simulink model "Shading_Fuzzy_single_phase_inverter"  (R2025a)
settings: Solver=ode23tb  StartTime=0.0  StopTime=2  FixedStep=1e-8  MaxStep=1e-5  RelTol=1e-4
values from neighbouring files (symbols this model uses):
  init_duty = 0.5    [generate_final_results.m]    (also in master_eval.m; params.m)
  sample_time_FLC = 0.005    [generate_final_results.m]    (also in master_eval.m; params.m)
  sample_time_mv_avg = 1e-4    (= 0.0001)    [generate_final_results.m]    (also in master_eval.m; params.m)
  temp = 25    [data_gen.m]    (also in generate_final_results.m; master_eval.m; params.m; shade_no_shade_graphs.m)
undefined symbols (not defined in the file or in its folder): DiscIntNeverNeededParam, irr
libraries: spsMosfetLib x5, spsSeriesRLCBranchLib x5, eeGeneralControl x3, spsCurrentMeasurementLib x2, spsFirstOrderFilterLib x2, slpidlib x2, simulink x2, spsVoltageMeasurementLib x2, spsACVoltageSourceLib x1, spsAlphaBetaZerotodq0Lib x1, spsDiodeLib x1, fuzblock x1
settings Model: Creator=gayathri  LastModifiedBy=harsh

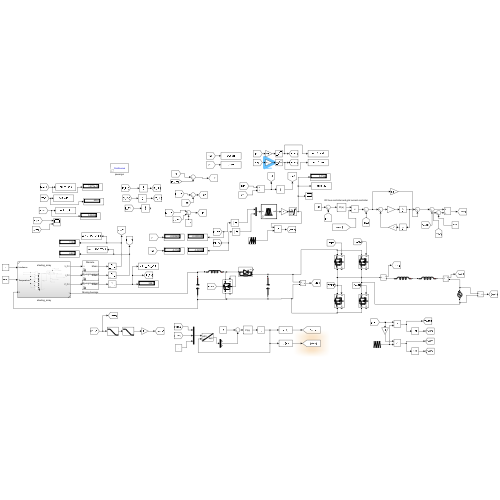
[thumbnail: Simulink's stored preview of the top-level diagram]
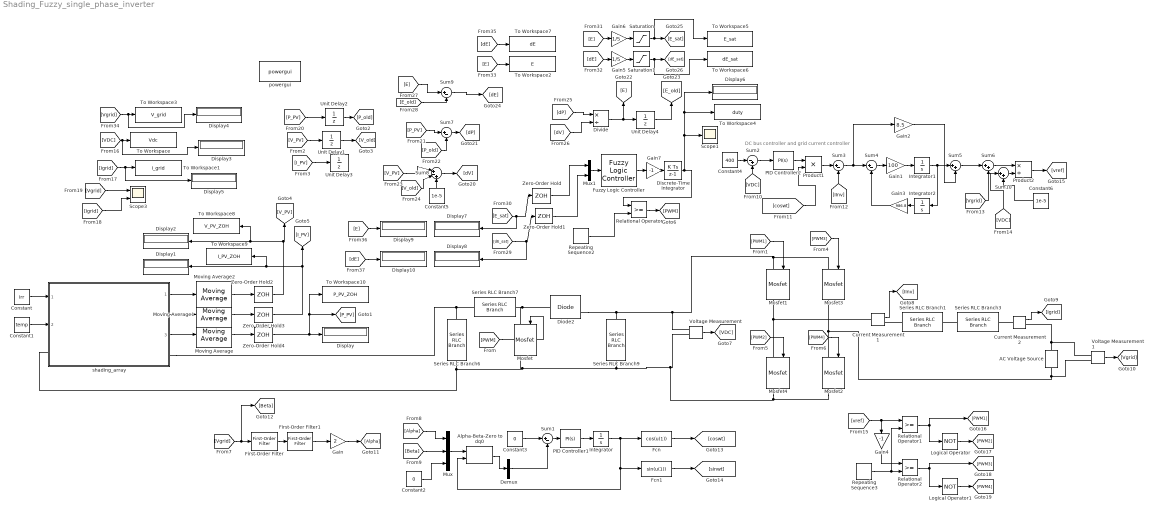
== system Shading_Fuzzy_single_phase_inverter ==
  note: DC bus controller and grid current controller
  AC Voltage Source : spsACVoltageSourceLib/AC Voltage Source  Amplitude=325  Phase=0  Frequency=50  SampleTime=0  Measurements=None  BusType=swing  Pref=10e3  Qref=0  Qmin=-inf  Qmax=+inf
  Alpha-Beta-Zero to dq0 : spsAlphaBetaZerotodq0Lib/Alpha-Beta-Zero to dq0  Alignment=90 degrees behind phase A axis
  Constant : Constant  Value=irr
  Constant1 : Constant  Value=temp
  Constant2 : Constant  Value=0
  Constant3 : Constant  Value=0
  Constant4 : Constant  Value=400
  Constant5 : Constant  Value=1e-5
  Constant6 : Constant  Value=1e-5
  Current Measurement1 : spsCurrentMeasurementLib/Current Measurement  PhasorSimulation=off  OutputType=Complex  PSBequivalent=0
  Current Measurement2 : spsCurrentMeasurementLib/Current Measurement  PhasorSimulation=off  OutputType=Complex  PSBequivalent=0
  Demux : Demux  Outputs=3
  Diode2 : spsDiodeLib/Diode  Ron=0.001  Lon=0  Vf=0.8  IC=0  UseSnubber=0  Rs=500  Cs=250e-9  Measurements=on
  Discrete-Time Integrator : DiscreteIntegrator  InitialCondition=init_duty  SampleTime=sample_time_FLC  LimitOutput=on  UpperSaturationLimit=0.9  LowerSaturationLimit=0.1  ICPrevOutput=DiscIntNeverNeededParam  ICPrevScaledInput=DiscIntNeverNeededParam
  Display{,1..10} (11 alike) : Display
  Divide : Product  Inputs=*/
  Fcn : Fcn  Expr=cos(u(1))
  Fcn1 : Fcn  Expr=sin(u(1))
  First-Order Filter : spsFirstOrderFilterLib/First-Order Filter  FilterType=Lowpass  Tc=1/(2*pi*50)  Ts=0  Initialize=off  Vac_Init=[0, 0, 60]  Vdc_Init=0  PlotResponse=off  FreqRange="[0,  200,  1]"
  First-Order Filter1 : spsFirstOrderFilterLib/First-Order Filter  FilterType=Lowpass  Tc=1/(2*pi*50)  Ts=0  Initialize=off  Vac_Init=[0, 0, 60]  Vdc_Init=0  PlotResponse=off  FreqRange="[0,  200,  1]"
  Fuzzy Logic Controller : fuzblock/Fuzzy Logic  Controller  FIS='fuzzy_mppt.fis'  OutputSampleNumber=101  DataType=double  UseLookupTable=off  NumBreakpoints=10  FuzzifiedInputs=off  RuleFiringStrengths=off  RuleOutputs=off  AggregatedOutputs=off  SimulateUsing=Interpreted execution  OutOfRangeInputValueMessage=warning  NoRuleFiredMessage=warning  EmptyOutputFuzzySetMessage=warning
  Gain : Gain  Gain=2
  Gain1 : Gain  Gain=100
  Gain2 : Gain  Gain=8.5
  Gain3 : Gain  Gain=986.8
  Gain4 : Gain  Gain=-1
  Gain5 : Gain  Gain=1/5
  Gain6 : Gain  Gain=1/5
  Gain7 : Gain  Gain=-1
  Integrator : Integrator
  Integrator1 : Integrator
  Integrator2 : Integrator
  Logical Operator : Logic  Operator=NOT  AllPortsSameDT=off  OutDataTypeStr=boolean
  Logical Operator1 : Logic  Operator=NOT  AllPortsSameDT=off  OutDataTypeStr=boolean
  Mosfet{,1..4} (5 alike) : spsMosfetLib/Mosfet  Ron=0.1  Lon=0  Rd=0.01  Vfd=0  IC=0  Rs=1e5  Cs=inf  Measurements=on
  Moving Average : eeGeneralControl/Moving Average  VariantControl=Variant1  LabelModeActiveChoice=Discrete  f=100  x0=0  BufferSize=8192  Ts=sample_time_mv_avg
      settings: LibrarySourceBlock=ee_sl_lib/General Control/Moving Average
  Moving Average1 : eeGeneralControl/Moving Average  VariantControl=Variant1  LabelModeActiveChoice=Discrete  f=100  x0=0  BufferSize=8192  Ts=sample_time_mv_avg
      settings: LibrarySourceBlock=ee_sl_lib/General Control/Moving Average
  Moving Average2 : eeGeneralControl/Moving Average  VariantControl=Variant1  LabelModeActiveChoice=Discrete  f=100  x0=0  BufferSize=8192  Ts=sample_time_mv_avg
      settings: LibrarySourceBlock=ee_sl_lib/General Control/Moving Average
  Mux : Mux  Inputs=3
  Mux1 : Mux  Inputs=2
  PID Controller1 : slpidlib/PID Controller  Controller=PI  Form=Parallel  TimeDomain=Continuous-time  UseExternalTs=off  SampleTime=-1  IntegratorMethod=Forward Euler  FilterMethod=Forward Euler  ControllerParametersSource=internal  P=10  I=5000  UseKiTs=off  D=0  UseExternalDerivativeSource=off  N=100  UseFilter=on  TunerSelectOption=Transfer Function Based (PID Tuner App)  InitialConditionSource=internal  InitialConditionForIntegrator=0  InitialConditionForFilter=0  DifferentiatorICPrevScaledInput=0  ExternalReset=none  TrackingMode=off  Kt=1  LimitOutput=off  SatLimitsSource=internal  UpperSaturationLimit=inf  LowerSaturationLimit=-inf  LinearizeAsGain=on  AntiWindupMode=none  Kb=1  LimitIntegrator=off  UpperIntegratorSaturationLimit=inf  LowerIntegratorSaturationLimit=-inf  POutMin=[]  POutMax=[]  IOutMin=[]  IOutMax=[]  DOutMin=[]  DOutMax=[]  NOutMin=[]  NOutMax=[]  SumOutMin=[]  SumOutMax=[]  SaturationOutMin=[]  SaturationOutMax=[]  PParamMin=[]  PParamMax=[]  IParamMin=[]  IParamMax=[]  DParamMin=[]  DParamMax=[]  NParamMin=[]  NParamMax=[]  KbParamMin=[]  KbParamMax=[]  KtParamMin=[]  KtParamMax=[]  KbOutMin=[]  KbOutMax=[]  KtOutMin=[]  KtOutMax=[]  IntegratorOutMin=[]  IntegratorOutMax=[]  FilterOutMin=[]  FilterOutMax=[]  SumI1OutMin=[]  SumI1OutMax=[]  SumI2OutMin=[]  SumI2OutMax=[]  SumI3OutMin=[]  SumI3OutMax=[]  SumI4OutMin=[]  SumI4OutMax=[]  SumDOutMin=[]  SumDOutMax=[]  DifferentiatorOutMin=[]  DifferentiatorOutMax=[]  FilterDiffOutCoefMin=[]  FilterDiffOutCoefMax=[]  ReciprocalOutMin=[]  ReciprocalOutMax=[]  SumDenOutMin=[]  SumDenOutMax=[]  SumNumOutMin=[]  SumNumOutMax=[]  DivideOutMin=[]  DivideOutMax=[]  UdiffTsProdOutMin=[]  UdiffTsProdOutMax=[]  NTsProdOutMin=[]  NTsProdOutMax=[]  UintegralTsProdOutMin=[]  UintegralTsProdOutMax=[]  UngainTsProdOutMin=[]  UngainTsProdOutMax=[]  ClampingZeroOutDataTypeStr=Inherit: Inherit via back propagation  ClampingZeroOutMin=[]  ClampingZeroOutMax=[]  FilterDenConstantOutDataTypeStr=Inherit: Inherit via back propagation  FilterDenConstantOutMin=[]  FilterDenConstantOutMax=[]  PCopyOutDataTypeStr=Inherit: Inherit via back propagation  PCopyOutMin=[]  PCopyOutMax=[]  NCopyOutDataTypeStr=Inherit: Inherit via back propagation  NCopyOutMin=[]  NCopyOutMax=[]  IntegratorContinuousStateAttributes=''  IntegratorStateMustResolveToSignalObject=off  IntegratorRTWStateStorageClass=Auto  FilterContinuousStateAttributes=''  FilterStateMustResolveToSignalObject=off  FilterRTWStateStorageClass=Auto  ParallelPVariant=InternalParameters  IdealPVariant=Disabled  IVariant=InternalParameters  DVariant=Disabled  IntegratorVariant=Continuous  SatVariant=Disabled  AWVariant=Passthrough  PCopyVariant=Disabled  TRVariant=Disabled  FdbkBlocksVariant=Forward  IdealPFdbkVariant=Disabled  SatFdbkVariant=Disabled  DerivativeFilterVariant=Disabled  NVariant=Disabled  NCopyVariant=Disabled_SignalSpec  FilterICVariant=Disabled  IntegratorICVariant=InternalICs  ExternalResetVariant=Disabled  TRSumVariant=Passthrough  SumFdbkVariant=Disabled  SumVariant=Sum_PI  TsampFilterVariant=InternalTs  TsampNgainVariant=Passthrough  TsampIntegralVariant=Disabled_SignalSpec  ExternalSaturationOutDataTypeStr=Inherit: Same as second input  DerivativeSourceVariant=Disabled  PreIntVariant=InternalPreInt
  PID Controller2 : slpidlib/PID Controller  Controller=PI  Form=Parallel  TimeDomain=Continuous-time  UseExternalTs=off  SampleTime=-1  IntegratorMethod=Forward Euler  FilterMethod=Forward Euler  ControllerParametersSource=internal  P=0.75  I=10  UseKiTs=off  D=0  UseExternalDerivativeSource=off  N=100  UseFilter=on  TunerSelectOption=Transfer Function Based (PID Tuner App)  InitialConditionSource=internal  InitialConditionForIntegrator=0  InitialConditionForFilter=0  DifferentiatorICPrevScaledInput=0  ExternalReset=none  TrackingMode=off  Kt=1  LimitOutput=off  SatLimitsSource=internal  UpperSaturationLimit=inf  LowerSaturationLimit=-inf  LinearizeAsGain=on  AntiWindupMode=none  Kb=1  LimitIntegrator=off  UpperIntegratorSaturationLimit=inf  LowerIntegratorSaturationLimit=-inf  POutMin=[]  POutMax=[]  IOutMin=[]  IOutMax=[]  DOutMin=[]  DOutMax=[]  NOutMin=[]  NOutMax=[]  SumOutMin=[]  SumOutMax=[]  SaturationOutMin=[]  SaturationOutMax=[]  PParamMin=[]  PParamMax=[]  IParamMin=[]  IParamMax=[]  DParamMin=[]  DParamMax=[]  NParamMin=[]  NParamMax=[]  KbParamMin=[]  KbParamMax=[]  KtParamMin=[]  KtParamMax=[]  KbOutMin=[]  KbOutMax=[]  KtOutMin=[]  KtOutMax=[]  IntegratorOutMin=[]  IntegratorOutMax=[]  FilterOutMin=[]  FilterOutMax=[]  SumI1OutMin=[]  SumI1OutMax=[]  SumI2OutMin=[]  SumI2OutMax=[]  SumI3OutMin=[]  SumI3OutMax=[]  SumI4OutMin=[]  SumI4OutMax=[]  SumDOutMin=[]  SumDOutMax=[]  DifferentiatorOutMin=[]  DifferentiatorOutMax=[]  FilterDiffOutCoefMin=[]  FilterDiffOutCoefMax=[]  ReciprocalOutMin=[]  ReciprocalOutMax=[]  SumDenOutMin=[]  SumDenOutMax=[]  SumNumOutMin=[]  SumNumOutMax=[]  DivideOutMin=[]  DivideOutMax=[]  UdiffTsProdOutMin=[]  UdiffTsProdOutMax=[]  NTsProdOutMin=[]  NTsProdOutMax=[]  UintegralTsProdOutMin=[]  UintegralTsProdOutMax=[]  UngainTsProdOutMin=[]  UngainTsProdOutMax=[]  ClampingZeroOutDataTypeStr=Inherit: Inherit via back propagation  ClampingZeroOutMin=[]  ClampingZeroOutMax=[]  FilterDenConstantOutDataTypeStr=Inherit: Inherit via back propagation  FilterDenConstantOutMin=[]  FilterDenConstantOutMax=[]  PCopyOutDataTypeStr=Inherit: Inherit via back propagation  PCopyOutMin=[]  PCopyOutMax=[]  NCopyOutDataTypeStr=Inherit: Inherit via back propagation  NCopyOutMin=[]  NCopyOutMax=[]  IntegratorContinuousStateAttributes=''  IntegratorStateMustResolveToSignalObject=off  IntegratorRTWStateStorageClass=Auto  FilterContinuousStateAttributes=''  FilterStateMustResolveToSignalObject=off  FilterRTWStateStorageClass=Auto  ParallelPVariant=InternalParameters  IdealPVariant=Disabled  IVariant=InternalParameters  DVariant=Disabled  IntegratorVariant=Continuous  SatVariant=Disabled  AWVariant=Passthrough  PCopyVariant=Disabled  TRVariant=Disabled  FdbkBlocksVariant=Forward  IdealPFdbkVariant=Disabled  SatFdbkVariant=Disabled  DerivativeFilterVariant=Disabled  NVariant=Disabled  NCopyVariant=Disabled_SignalSpec  FilterICVariant=Disabled  IntegratorICVariant=InternalICs  ExternalResetVariant=Disabled  TRSumVariant=Passthrough  SumFdbkVariant=Disabled  SumVariant=Sum_PI  TsampFilterVariant=InternalTs  TsampNgainVariant=Passthrough  TsampIntegralVariant=Disabled_SignalSpec  ExternalSaturationOutDataTypeStr=Inherit: Same as second input  DerivativeSourceVariant=Disabled  PreIntVariant=InternalPreInt
  Product1 : Product
  Product2 : Product  Inputs=*/
  Relational Operator : RelationalOperator  OutDataTypeStr=boolean  RndMeth=Simplest  InputSameDT=off
  Relational Operator1 : RelationalOperator  OutDataTypeStr=boolean  RndMeth=Simplest  InputSameDT=off
  Relational Operator2 : RelationalOperator  OutDataTypeStr=boolean  RndMeth=Simplest  InputSameDT=off
  Repeating Sequence2 : simulink/Sources/Repeating Sequence  rep_seq_t=[0 0.0002]  rep_seq_y=[0 1]
  Repeating Sequence3 : simulink/Sources/Repeating Sequence  rep_seq_t=[0 0.00005 0.0001]  rep_seq_y=[-1 1 -1]
  Saturation : Saturate  UpperLimit=1  LowerLimit=-1  LinearizeAsGain=off
  Saturation1 : Saturate  UpperLimit=1  LowerLimit=-1  LinearizeAsGain=off
  Scope1 : Scope
      settings: ActiveDisplayYMinimum=0.04930916133207007  ActiveDisplayYMaximum=0.55621754801136958
  Scope3 : Scope  NumInputPorts=2
      settings: ActiveDisplayYMinimum=-406.25  ActiveDisplayYMaximum=406.25  DataLoggingVariableName=ScopeData3
  Series RLC Branch1 : spsSeriesRLCBranchLib/Series RLC Branch  LConnTagsString=__new0  RConnTagsString=__new0  BranchType=L  Resistance=0.0001  Inductance=4.06e-3  SetiL0=off  InitialCurrent=0  Capacitance=1000e-6  Setx0=off  InitialVoltage=0  Measurements=None
  Series RLC Branch3 : spsSeriesRLCBranchLib/Series RLC Branch  LConnTagsString=__new0  RConnTagsString=__new0  BranchType=L  Resistance=0.0001  Inductance=4.35e-3  SetiL0=off  InitialCurrent=0  Capacitance=1000e-6  Setx0=off  InitialVoltage=0  Measurements=None
  Series RLC Branch6 : spsSeriesRLCBranchLib/Series RLC Branch  LConnTagsString=__new0  RConnTagsString=__new0  BranchType=C  Resistance=0.0001  Inductance=1e-3  SetiL0=off  InitialCurrent=0  Capacitance=500e-6  Setx0=off  InitialVoltage=40  Measurements=None
  Series RLC Branch7 : spsSeriesRLCBranchLib/Series RLC Branch  LConnTagsString=__new0  RConnTagsString=__new0  BranchType=L  Resistance=0.0001  Inductance=20e-3  SetiL0=off  InitialCurrent=0  Capacitance=1000e-6  Setx0=off  InitialVoltage=0  Measurements=None
  Series RLC Branch9 : spsSeriesRLCBranchLib/Series RLC Branch  LConnTagsString=__new0  RConnTagsString=__new0  BranchType=C  Resistance=0.0001  Inductance=1.45e-3  SetiL0=off  InitialCurrent=0  Capacitance=3000e-6  Setx0=off  InitialVoltage=0  Measurements=None
  Sum{1,3..4,7,9} (5 alike) : Sum  Inputs=|+-
  Sum10 : Sum  Inputs=|++
  Sum2 : Sum  Inputs=|-+
  Sum5 : Sum  Inputs=|++
  Sum6 : Sum  Inputs=|++
  Sum8 : Sum  Inputs=|+-+
  To Workspace : ToWorkspace  VariableName=Vdc  SampleTime=-1
  To Workspace1 : ToWorkspace  VariableName=I_grid  SampleTime=-1
  To Workspace10 : ToWorkspace  VariableName=P_PV_ZOH  SampleTime=-1
  To Workspace2 : ToWorkspace  VariableName=E  SampleTime=-1
  To Workspace3 : ToWorkspace  VariableName=V_grid  SampleTime=-1
  To Workspace4 : ToWorkspace  VariableName=duty  SampleTime=-1
  To Workspace5 : ToWorkspace  VariableName=E_sat  SampleTime=-1
  To Workspace6 : ToWorkspace  VariableName=dE_sat  SampleTime=-1
  To Workspace7 : ToWorkspace  VariableName=dE  SampleTime=-1
  To Workspace8 : ToWorkspace  VariableName=V_PV_ZOH  SampleTime=-1
  To Workspace9 : ToWorkspace  VariableName=I_PV_ZOH  SampleTime=-1
  Unit Delay{1..4} (4 alike) : UnitDelay  SampleTime=sample_time_FLC  HasFrameUpgradeWarning=on
  Voltage Measurement : spsVoltageMeasurementLib/Voltage Measurement  PhasorSimulation=off  OutputType=Complex  PSBequivalent=0
  Voltage Measurement1 : spsVoltageMeasurementLib/Voltage Measurement  PhasorSimulation=off  OutputType=Complex  PSBequivalent=0
  Zero-Order Hold{,1..4} (5 alike) : ZeroOrderHold  SampleTime=sample_time_FLC
  powergui : sps_lib/powergui  Priority=1  SimulationMode=Continuous  SampleTime=1e-6  frequency=60  Iterations=50  frequencyindice=0  Pbase=100e6  ErrMax=1e-4  UnitsV=kV  UnitsW=MW  buscounter=0  FunctionMessages=off  echomessages=off  EnableUseOfTLC=off  CurrentSourceSwitches=off  DisableSnubberDevices=off  DisableRonSwitches=off  DisableVfSwitches=off  DisplayEquations=off  AutomaticDiscreteSolvers=off  SolverType=Tustin/Backward Euler (TBE)  Interpol=off  ExternalGateDelay=off  methode=off  Ts=100  x0status=blocks  SPID=on  SwTol=0  HookPort=off  NonlinearTolerance=1e-4  nMaxIteration=100  ContinueOnMaxIteration=off  RestoreLinks=warning  ResistiveCurrentMeasurement=off  Frange=[0:2:500]  Ylog=off  Xlog=on  ShowGrid=off  save=off  variable=ZData  structure=0  ZoomFFT=off  StartTime=0.0  cycles=1  DisplayStyle=1  fundamental=60  FreqAxis=off  MaxFrequency=1000  frequencyindicesteady=1  RmsSteady=1  display=off
  shading_array : Subsystem  ReferencedSubsystem=shading_array
  wires:
  [V_PV] -> Unit Delay1/1
  [I_PV] -> Unit Delay3/1
  Unit Delay1/1 -> [V_old]
  Repeating Sequence2/1 -> Relational Operator/2
  Relational Operator/1 -> [PWM]
  shading_array/3 -> Moving Average/1
  Voltage Measurement/1 -> [VDC]
  shading_array/1 -> Moving Average2/1
  [PWM] -> Mosfet/1
  [PWM1] -> Mosfet1/1
  [PWM3] -> Mosfet3/1
  [PWM2] -> Mosfet4/1
  [PWM4] -> Mosfet2/1
  Current Measurement1/1 -> [IInv]
  Current Measurement2/1 -> [Igrid]
  Voltage Measurement1/1 -> [Vgrid]
  [Vgrid] -> [Beta], First-Order Filter/1
  First-Order Filter/1 -> First-Order Filter1/1
  First-Order Filter1/1 -> Gain/1
  Gain/1 -> [Alpha]
  [Alpha] -> Mux/1
  [Beta] -> Mux/2
  Constant2/1 -> Mux/3
  Mux/1 -> Alpha-Beta-Zero to dq0/1
  Alpha-Beta-Zero to dq0/1 -> Demux/1
  Demux/2 -> Sum1/2
  Constant3/1 -> Sum1/1
  Sum1/1 -> PID Controller1/1
  PID Controller1/1 -> Integrator/1
  Integrator/1 -> Fcn/1, Fcn1/1, Alpha-Beta-Zero to dq0/2
  Fcn/1 -> [coswt]
  Fcn1/1 -> [sinwt]
  Constant4/1 -> Sum2/1
  [VDC] -> Sum2/2
  Sum2/1 -> PID Controller2/1
  PID Controller2/1 -> Product1/1
  [coswt] -> Product1/2
  Product1/1 -> Sum3/1
  [IInv] -> Sum3/2
  Sum3/1 -> Gain2/1, Sum4/1
  Sum4/1 -> Gain1/1
  Gain1/1 -> Integrator1/1
  Gain2/1 -> Sum5/2
  Integrator1/1 -> Integrator2/1, Sum5/1
  Integrator2/1 -> Gain3/1
  Gain3/1 -> Sum4/2
  Sum5/1 -> Sum6/1
  [Vgrid] -> Sum6/2
  Sum6/1 -> Product2/1
  Product2/1 -> [vref]
  [vref] -> Gain4/1, Relational Operator1/1
  Gain4/1 -> Relational Operator2/1
  Repeating Sequence3/1 -> Relational Operator1/2, Relational Operator2/2
  Relational Operator2/1 -> [PWM3], Logical Operator1/1
  Relational Operator1/1 -> [PWM1], Logical Operator/1
  Logical Operator/1 -> [PWM2]
  Logical Operator1/1 -> [PWM4]
  [VDC] -> Display3/1, To Workspace/1
  [Igrid] -> Display5/1, To Workspace1/1
  [Vgrid] -> Scope3/1
  [Igrid] -> Scope3/2
  [P_PV] -> Unit Delay2/1
  Unit Delay2/1 -> [P_old]
  [P_PV] -> Sum7/1
  [P_old] -> Sum7/2
  [V_PV] -> Sum8/1
  [V_old] -> Sum8/2
  Constant5/1 -> Sum8/3
  Sum8/1 -> [dV]
  Sum7/1 -> [dP]
  [dP] -> Divide/1
  [dV] -> Divide/2
  Divide/1 -> Unit Delay4/1, [E]
  Unit Delay4/1 -> [E_old]
  [E] -> Sum9/1
  [E_old] -> Sum9/2
  Sum9/1 -> [dE]
  Mux1/1 -> Fuzzy Logic Controller/1
  Discrete-Time Integrator/1 -> Display6/1, To Workspace4/1, Scope1/1, Relational Operator/1
  [E] -> Gain6/1
  [dE] -> Gain5/1
  Gain5/1 -> Saturation1/1
  Gain6/1 -> Saturation/1
  Fuzzy Logic Controller/1 -> Gain7/1
  Gain7/1 -> Discrete-Time Integrator/1
  shading_array/2 -> Moving Average1/1
  Constant/1 -> shading_array/1
  Constant1/1 -> shading_array/2
  [Vgrid] -> Display4/1, To Workspace3/1
  Saturation/1 -> To Workspace5/1, [E_sat]
  Saturation1/1 -> To Workspace6/1, [dE_sat]
  Sum10/1 -> Product2/2
  [VDC] -> Sum10/1
  Constant6/1 -> Sum10/2
  [E_sat] -> Display7/1, Zero-Order Hold/1
  Zero-Order Hold/1 -> Mux1/1
  Zero-Order Hold1/1 -> Mux1/2
  [dE_sat] -> Zero-Order Hold1/1, Display8/1
  [E] -> To Workspace2/1
  [dE] -> To Workspace7/1
  [E] -> Display9/1
  [dE] -> Display10/1
  Moving Average/1 -> Zero-Order Hold4/1
  Moving Average1/1 -> Zero-Order Hold3/1
  Moving Average2/1 -> Zero-Order Hold2/1
  Zero-Order Hold2/1 -> To Workspace8/1, Display2/1, [V_PV]
  Zero-Order Hold3/1 -> [I_PV], To Workspace9/1, Display1/1
  Zero-Order Hold4/1 -> To Workspace10/1, [P_PV], Display/1
  connections:
  Series RLC Branch7/RConn1 -- shading_array/RConn1 -- Series RLC Branch6/LConn1
  Diode2/LConn1 -- Series RLC Branch7/LConn1 -- Mosfet/LConn1
  Diode2/RConn1 -- Series RLC Branch9/LConn1 -- Mosfet3/LConn1 -- Mosfet1/LConn1 -- Voltage Measurement/LConn1
  Series RLC Branch9/RConn1 -- Mosfet2/RConn1 -- Mosfet4/RConn1 -- Voltage Measurement/LConn2 -- Mosfet/RConn1 -- shading_array/LConn1 -- Series RLC Branch6/RConn1
  Mosfet4/LConn1 -- Current Measurement1/LConn1 -- Mosfet1/RConn1
  Mosfet2/LConn1 -- Voltage Measurement1/LConn2 -- AC Voltage Source/LConn1 -- Mosfet3/RConn1
  Series RLC Branch3/RConn1 -- Series RLC Branch1/LConn1
  Series RLC Branch1/RConn1 -- Current Measurement1/RConn1
  Current Measurement2/LConn1 -- Series RLC Branch3/LConn1
  AC Voltage Source/RConn1 -- Current Measurement2/RConn1 -- Voltage Measurement1/LConn1
